simulink model "eha_model"  (R2015b)
settings: Solver=VariableStepAuto  StartTime=0.0  StopTime=10.0  RelTol=1e-3
values from neighbouring files (symbols this model uses):
  A = [ 1 0.001 0; 0 1 0.001; -557.02 -28.616 0.9418]    [eha_w_kalman_filter.m]
  B = [0 0 557.02]'    [eha_w_kalman_filter.m]
  C = H    [eha_w_kalman_filter.m]
  K = place(A,B,poles)    [eha_w_kalman_filter.m]    (also in run_eha.m)
  L = L'    [run_eha.m]
  Nbar = rscale(sys,K)    [eha_w_kalman_filter.m]    (also in run_eha.m)
settings Model: Creator=Nicholas  LastModifiedBy=Nicholas

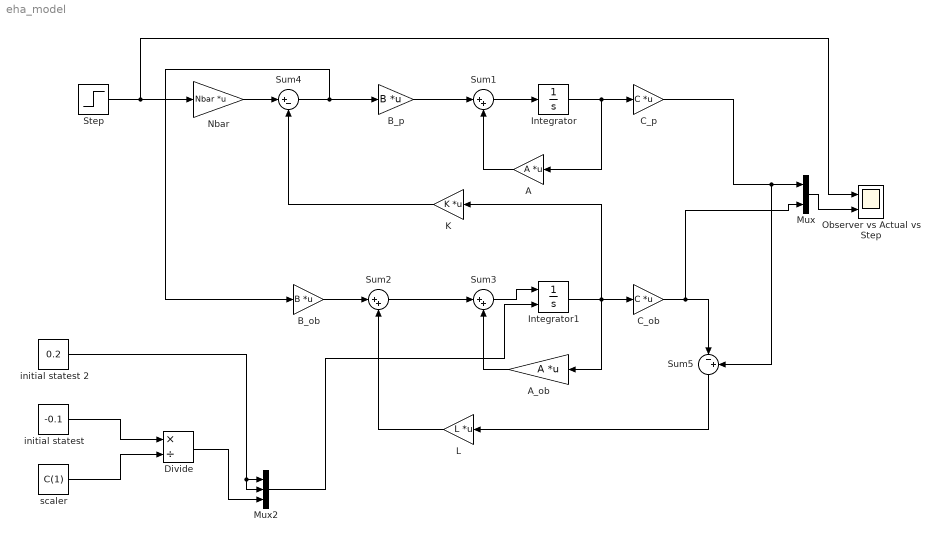
== system eha_model ==
  A : Gain  Gain=A  Multiplication=Matrix(K*u)
  A_ob : Gain  Gain=A  Multiplication=Matrix(K*u)
  B_ob : Gain  Gain=B  Multiplication=Matrix(K*u)
  B_p : Gain  Gain=B  Multiplication=Matrix(K*u)
  C_ob : Gain  Gain=C  Multiplication=Matrix(K*u)
  C_p : Gain  Gain=C  Multiplication=Matrix(K*u)
  Divide : Product  Inputs=*/
  Integrator : Integrator
  Integrator1 : Integrator  InitialConditionSource=external  InitialCondition=[0 0 0]
  K : Gain  Gain=K  Multiplication=Matrix(K*u)
  L : Gain  Gain=L  Multiplication=Matrix(K*u)
  Mux : Mux  Inputs=2
  Mux2 : Mux  Inputs=3
  Nbar : Gain  Gain=Nbar  Multiplication=Matrix(K*u)
  "Observer vs Actual vs Step " : Scope  NumInputPorts=2
  Step : Step  SampleTime=0
  Sum1 : Sum  Inputs=|++
  Sum2 : Sum  Inputs=|++
  Sum3 : Sum  Inputs=|++
  Sum4 : Sum  Inputs=|+-
  Sum5 : Sum  Inputs=|-+
  "initial statest " : Constant  Value=-0.1
  initial statest 2 : Constant  Value=0.2
  scaler : Constant  Value=C(1)
  wires:
  A/1 -> Sum1/2
  Sum1/1 -> Integrator/1
  Integrator/1 -> A/1, C_p/1
  L/1 -> Sum2/2
  Sum2/1 -> Sum3/1
  A_ob/1 -> Sum3/2
  Sum3/1 -> Integrator1/1
  Integrator1/1 -> K/1, C_ob/1, A_ob/1
  C_ob/1 -> Sum5/1, Mux/2
  B_ob/1 -> Sum2/1
  B_p/1 -> Sum1/1
  K/1 -> Sum4/2
  Sum4/1 -> B_ob/1, B_p/1
  Sum5/1 -> L/1
  Step/1 -> "Observer vs Actual vs Step "/1, Nbar/1
  C_p/1 -> Sum5/2, Mux/1
  Nbar/1 -> Sum4/1
  Mux/1 -> "Observer vs Actual vs Step "/2
  "initial statest "/1 -> Divide/1
  scaler/1 -> Divide/2
  Divide/1 -> Mux2/3
  initial statest 2/1 -> Mux2/2, Mux2/1
  Mux2/1 -> Integrator1/2
